simulink model "labc2_arduino_22_julho"  (R2023a)
settings: Solver=VariableStepAuto  StartTime=0.0  StopTime=5  RelTol=1e-3
values from neighbouring files (symbols this model uses):
  A = [-Ra/La -kg/La/kt; ka*kt/J -f/J]    [labc2_p2_final.m]    (also in robusto2_lc2.m = [[ -113.5203 -34.3792];[27.0249 -0.3312]]; robusto_labc2.m = [[ -113.5203 -34.3792];[27.0249 -0.3312]])
  b = [1/La;0]    [labc2_p2_final.m]    (also in robusto2_lc2.m = [46.6079 0]'; robusto_labc2.m = [46.6079 0]')
  c = [0 1]    [labc2_p2_final.m]    (also in robusto2_lc2.m; robusto_labc2.m)
  ki = k_total(3)    [labc2_p2_final.m]    (also in robusto2_lc2.m = k_robusto(end))
  kt = 0.1470    (= 0.147)    [labc2_p2_final.m]
  kt_ee = place(A, b, polos)    [labc2_p2_final.m]    (also in robusto2_lc2.m = k_robusto(1:2); robusto_labc2.m)
  L = place(A', c', p_obs)'    [robusto2_lc2.m]
  media4 = mean(d4.C4InV)    [labc2_p2_final.m]
undefined symbols (not defined in the file or in its folder): ganho_amppot, ganho_dt
settings Model: Creator=wesle  LastModifiedBy=wesle

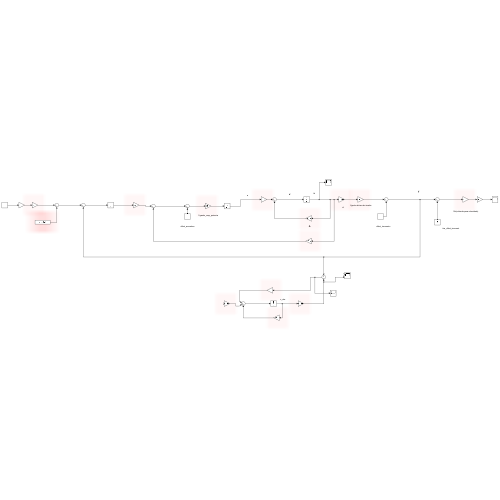
[thumbnail: Simulink's stored preview of the top-level diagram]
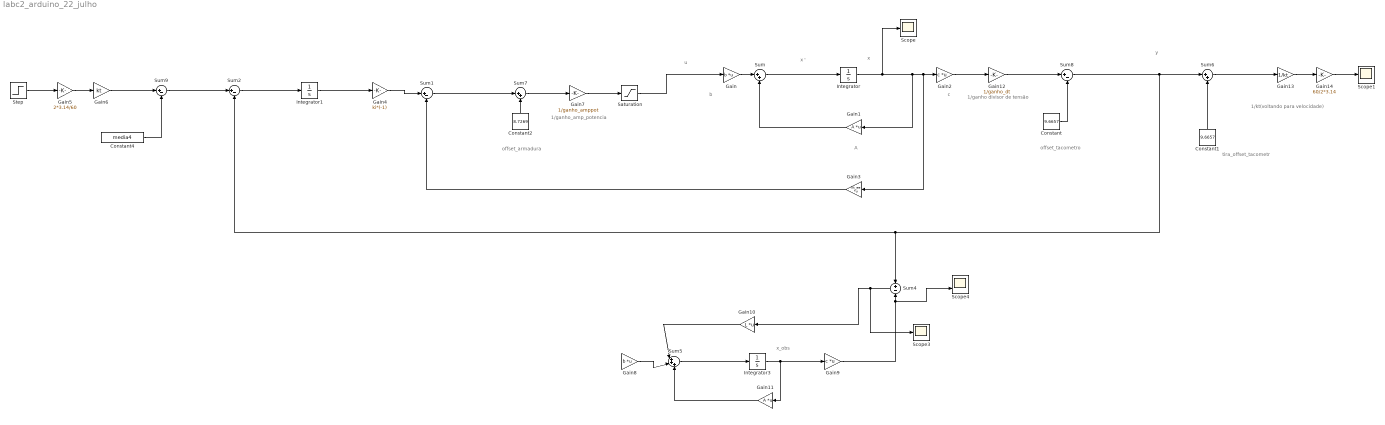
== system labc2_arduino_22_julho ==
  note: 1/kt(voltando para velocidade)
  note: 1/ganho divisor de tensão
  note: 1/ganho_amp_potencia
  note: u
  note: offset_armadura
  note: tira_offset_tacometr
  note: offset_tacometro
  note: x_obs
  note: b
  note: c
  note: A
  note: x '
  note: x
  note: y
  Constant : Constant  Value=9.6657
  Constant1 : Constant  Value=9.6657
  Constant2 : Constant  Value=8.7269
  Constant4 : Constant  Value=media4
  Gain : Gain  Gain=b  Multiplication=Matrix(K*u) (u vector)
  Gain1 : Gain  Gain=A  Multiplication=Matrix(K*u) (u vector)
  Gain10 : Gain  Gain=L  Multiplication=Matrix(K*u)
  Gain11 : Gain  Gain=A  Multiplication=Matrix(K*u) (u vector)
  Gain12 : Gain  Gain=1/ganho_dt
  Gain13 : Gain  Gain=1/kt
  Gain14 : Gain  Gain=60/2*3.14
  Gain2 : Gain  Gain=c  Multiplication=Matrix(K*u) (u vector)
  Gain3 : Gain  Gain=kt_ee  Multiplication=Matrix(K*u) (u vector)
  Gain4 : Gain  Gain=ki*(-1)
  Gain5 : Gain  Gain=2*3.14/60
  Gain6 : Gain  Gain=kt
  Gain7 : Gain  Gain=1/ganho_amppot
  Gain8 : Gain  Gain=b  Multiplication=Matrix(K*u) (u vector)
  Gain9 : Gain  Gain=c  Multiplication=Matrix(K*u) (u vector)
  Integrator : Integrator
  Integrator1 : Integrator
  Integrator3 : Integrator
  Saturation : Saturate
  Scope : Scope
  Scope1 : Scope
  Scope3 : Scope
  Scope4 : Scope  NumInputPorts=2
  Step : Step  SampleTime=0
  Sum : Sum  Inputs=|++
  Sum{1..2,8..9} (4 alike) : Sum  Inputs=|+-
  Sum4 : Sum  Inputs=+-
  Sum5 : Sum  Inputs=|+++
  Sum6 : Sum  Inputs=|++
  Sum7 : Sum  Inputs=|++
  wires:
  Sum/1 -> Integrator/1
  Gain/1 -> Sum/1
  Gain1/1 -> Sum/2
  Integrator/1 -> Scope/1, Gain1/1, Gain3/1, Gain2/1
  Gain3/1 -> Sum1/2
  Step/1 -> Gain5/1
  Sum2/1 -> Integrator1/1
  Integrator1/1 -> Gain4/1
  Gain4/1 -> Sum1/1
  Integrator3/1 -> Gain11/1, Gain9/1
  Gain8/1 -> Sum5/2
  Sum5/1 -> Integrator3/1
  Gain11/1 -> Sum5/3
  Gain9/1 -> Scope4/2, Sum4/2
  Sum4/1 -> Scope3/1, Gain10/1
  Gain10/1 -> Sum5/1
  Gain2/1 -> Gain12/1
  Constant/1 -> Sum8/2
  Sum8/1 -> Sum4/1, Sum2/2, Sum6/1
  Constant1/1 -> Sum6/2
  Constant2/1 -> Sum7/2
  Sum7/1 -> Gain7/1
  Saturation/1 -> Gain/1
  Gain5/1 -> Gain6/1
  Gain6/1 -> Sum9/1
  Constant4/1 -> Sum9/2
  Sum9/1 -> Sum2/1
  Sum1/1 -> Sum7/1
  Gain7/1 -> Saturation/1
  Gain12/1 -> Sum8/1
  Sum6/1 -> Gain13/1
  Gain13/1 -> Gain14/1
  Gain14/1 -> Scope1/1
